simulink model "CC_Flight_Simulation"  (R2026a)
settings: Solver=ode45  StopTime=120
InitFcn:
  | %%% Sensor with 3D measurement
  | % Define elements
  | elems(1) = Simulink.BusElement;
  | elems(1).Name = 'meas';
  | elems(1).Dimensions = 3;
  | elems(1).DataType = 'double';
  | elems(2) = Simulink.BusElement;
  | elems(2).Name = 'status';
  | elems(2).Dimensions = 1;
  | elems(2).DataType = 'boolean';
  | % Create bus
  | Sensor3DBus = Simulink.Bus;
  | Sensor3DBus.Elements = elems;
  | 
  | %%% Sensor with 1D measurement
  | % Define elements
  | elems(1) = Simulink.BusElement;
  | elems(1).Name = 'meas';
  | elems(1).Dimensions = 1;
  | elems(1).DataType = 'double';
  | elems(2) = Simulink.BusElement;
  | elems(2).Name = 'status';
  | elems(2).Dimensions = 1;
  | elems(2).DataType = 'boolean';
  | % Create bus
  | Sensor1DBus = Simulink.Bus;
  | Sensor1DBus.Elements = elems;
settings Model: SimulationMode=accelerator  Creator=bruno  LastModifiedBy=trist
settings OptimizationCC: GainParamInheritBuiltInType=on  UseFloatMulNetSlope=on  InlineInvariantSignals=on  EfficientFloat2IntCast=on
settings DebuggingCC: ArrayBoundsChecking=warning  MergeDetectMultiDrivingBlocksExec=warning  CheckMatrixSingularityMsg=warning  SFcnCompatibilityMsg=warning  UniqueDataStoreMsg=warning
settings HardwareCC: ProdBitPerLong=64.0  ProdHWDeviceType=AMD->x86-64 (Linux 64)
settings ModelReferenceCC: EnableParallelModelReferenceBuilds=on
settings SFSimCC: SimTargetLang=C++
settings RTWCC: Toolchain=Simulink Real-Time Linux x64 Remote Build Toolchain  BuildConfiguration=Faster Runs  TargetLang=C++  CheckMdlBeforeBuild=Warning
settings GRTTargetCC: TargetLangStandard=C++11 (ISO)  MatFileLogging=off  CodeInterfacePackaging=C++ class  SupportNonFinite=off

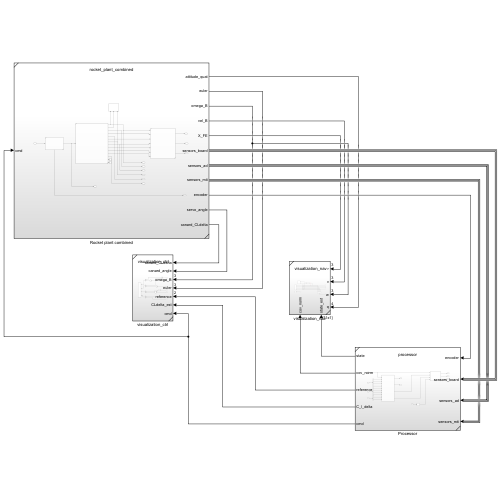
[thumbnail: Simulink's stored preview of the top-level diagram]
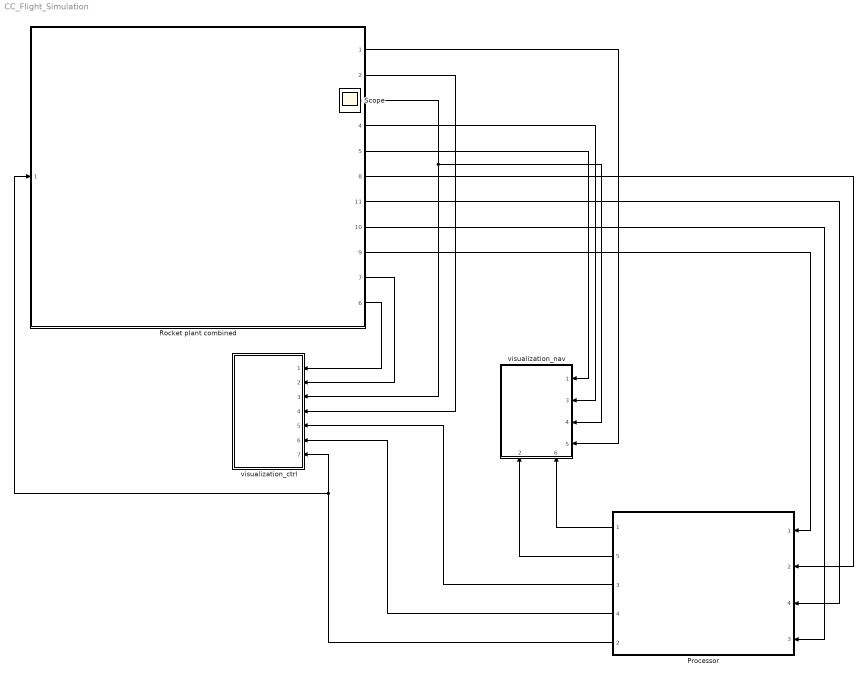
== system CC_Flight_Simulation ==
  Processor : Subsystem  ReferencedSubsystem=processor
      settings: PortSchema="{\"entries\":[{\"content\":{\"sides\":[{\"content\":{\"connectorIds\":[\"In1\",\"In2\",\"In4\",\"In3\"]},\"type\":\"ConnectorPlacement.EquallySpacedRectSide\",\"uuid\":\"3a8674be-3010-4d68-a33c-3eead0b8fa7c\"},{\"content\":{\"connectorIds\":[\"Out1\",\"Out5\",\"Out3\",\"Out4\",\"Out2\"],\"side\":\"RIGHT\"},\"type\":\"ConnectorPlacement.EquallySpacedRectSide\",\"uuid\":\"adad2a77-0efa-48c4-a551-5f502a84ce9d\"},{\"content\":{\"side\":\"TOP\"},\"type\":\"ConnectorPlacement.EquallySpacedRectSide\",\"uuid\":\"86d43adf-3710-4d07-a3fc-1076e1b690c3\"}]},\"type\":\"ConnectorPlacement.EquallySpacedConnector\",\"uuid\":\"03723af2-c1ac-4c1d-a4bb-0b905c3a6fdb\"}],\"packageUris\":[\"http://schema.mathworks.com/mf0/Connector/R2020b\"],\"version\":\"1.0\"}"
  Rocket plant combined : Subsystem  ReferencedSubsystem=rocket_plant_combined
      settings: PortSchema="{\"entries\":[{\"content\":{\"sides\":[{\"content\":{\"connectorIds\":[\"In1\"]},\"type\":\"ConnectorPlacement.EquallySpacedRectSide\",\"uuid\":\"b1d5c63c-66b0-4e52-a383-d076c7e4c195\"},{\"content\":{\"connectorIds\":[\"Out1\",\"Out2\",\"Out3\",\"Out4\",\"Out5\",\"Out8\",\"Out11\",\"Out10\",\"Out9\",\"Out7\",\"Out6\"],\"side\":\"RIGHT\"},\"type\":\"ConnectorPlacement.EquallySpacedRectSide\",\"uuid\":\"83da6c70-f7e5-4234-84e8-1f2c400394e6\"},{\"content\":{\"side\":\"TOP\"},\"type\":\"ConnectorPlacement.EquallySpacedRectSide\",\"uuid\":\"ef6370c9-9eee-494c-b1b6-fc765bebd62f\"}]},\"type\":\"ConnectorPlacement.EquallySpacedConnector\",\"uuid\":\"bbd76b48-4586-46ab-aeda-f955cbd51297\"}],\"packageUris\":[\"http://schema.mathworks.com/mf0/Connector/R2020b\"],\"version\":\"1.0\"}"
  visualization_ctrl : Subsystem  ReferencedSubsystem=visualization_ctrl
  visualization_nav : Subsystem  ReferencedSubsystem=visualization_nav
      settings: PortSchema="{\"entries\":[{\"content\":{\"sides\":[{\"content\":{\"connectorIds\":[\"In1\",\"In3\",\"In4\",\"In5\"]},\"type\":\"ConnectorPlacement.EquallySpacedRectSide\",\"uuid\":\"dc5fb855-67c6-44f2-b840-f485865d62e2\"},{\"content\":{\"side\":\"RIGHT\"},\"type\":\"ConnectorPlacement.EquallySpacedRectSide\",\"uuid\":\"f011a5d6-ba81-4cae-9458-00e11c499556\"},{\"content\":{\"side\":\"TOP\"},\"type\":\"ConnectorPlacement.EquallySpacedRectSide\",\"uuid\":\"2cb02a95-4340-4437-bf5a-0250095828b1\"},{\"content\":{\"connectorIds\":[\"In6\",\"In2\"],\"side\":\"BOTTOM\"},\"type\":\"ConnectorPlacement.EquallySpacedRectSide\",\"uuid\":\"f99cf30a-31eb-400e-ba65-b3afbbabbc8d\"}]},\"type\":\"ConnectorPlacement.EquallySpacedConnector\",\"uuid\":\"1a89fa10-7481-4e31-a831-abb3dd053fbf\"}],\"packageUris\":[\"http://schema.mathworks.com/mf0/Connector/R2020b\"],\"version\":\"1.0\"}"
  Scope : Scope
      settings: ActiveDisplayYMinimum=9.79326  ActiveDisplayYMaximum=9.80609
  wires:
  Processor/1 -> visualization_nav/6
  Processor/2 -> visualization_ctrl/7, Rocket plant combined/1
  Rocket plant combined/9 -> Processor/1
  Rocket plant combined/1 -> visualization_nav/5
  Rocket plant combined/2 -> visualization_ctrl/4
  Rocket plant combined/3 -> visualization_nav/4, visualization_ctrl/3
  Rocket plant combined/4 -> visualization_nav/3
  Rocket plant combined/5 -> visualization_nav/1
  Processor/3 -> visualization_ctrl/5
  Processor/4 -> visualization_ctrl/6
  Rocket plant combined/7 -> visualization_ctrl/2
  Rocket plant combined/6 -> visualization_ctrl/1
  Rocket plant combined/8 -> Processor/2
  Rocket plant combined/10 -> Processor/3
  Rocket plant combined/11 -> Processor/4
  Processor/5 -> visualization_nav/2
